simulink model "astr"  (R2017b)
settings: Solver=VariableStepAuto  StartTime=0.0  StopTime=10.0  RelTol=1e-3
undefined symbols (not defined in the file): Cube, mu_s
settings Model: Creator=hazr_sh  LastModifiedBy=shriyahazra

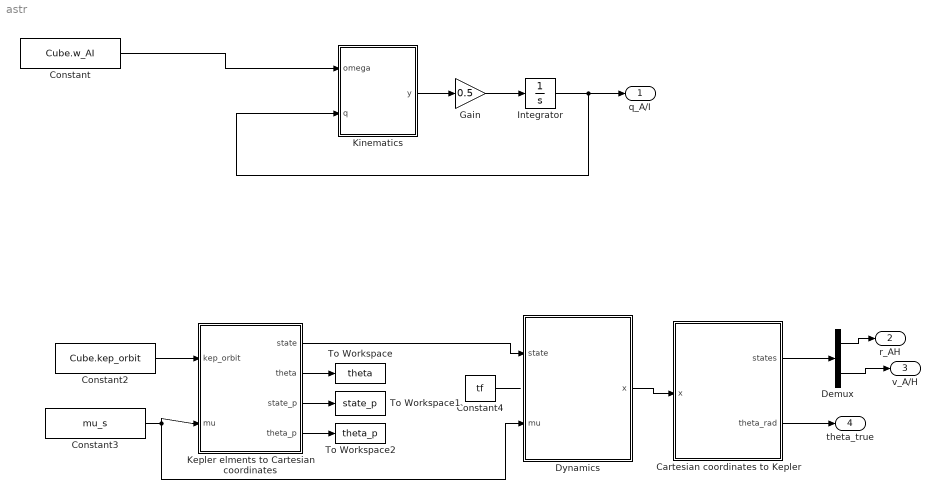
== system astr ==
  Cartesian coordinates to Kepler : MATLAB Function  TreatAsAtomicUnit=on
  Constant : Constant  Value=Cube.w_AI  VectorParams1D=off
  Constant2 : Constant  Value=Cube.kep_orbit  VectorParams1D=off
  Constant3 : Constant  Value=mu_s
  Constant4 : Constant  Value=tf
  Demux : Demux  Outputs=2
  Dynamics : MATLAB Function  TreatAsAtomicUnit=on
  Gain : Gain  Gain=0.5
  Integrator : Integrator  InitialCondition=[0 0 0 0]
  Kepler elments to Cartesian coordinates : MATLAB Function  TreatAsAtomicUnit=on
  Kinematics : MATLAB Function  TreatAsAtomicUnit=on
  To Workspace : ToWorkspace  VariableName=theta  SampleTime=-1
  To Workspace1 : ToWorkspace  VariableName=state_p  SampleTime=-1
  To Workspace2 : ToWorkspace  VariableName=theta_p  SampleTime=-1
  q_A/I : Outport
  r_AH : Outport  Port=2
  v_A/H : Outport  Port=3
  theta_true : Outport  Port=4
  wires:
  Kepler elments to Cartesian coordinates/3(state_p) -> To Workspace1/1
  Kepler elments to Cartesian coordinates/2(theta) -> To Workspace/1
  Dynamics/1(x) -> Cartesian coordinates to Kepler/1(x)
  Gain/1 -> Integrator/1
  Constant2/1 -> Kepler elments to Cartesian coordinates/1(kep_orbit)
  Demux/2 -> v_A/H/1
  Constant4/1 -> ?
  Demux/1 -> r_AH/1
  Cartesian coordinates to Kepler/1(states) -> Demux/1
  Constant3/1 -> Kepler elments to Cartesian coordinates/2(mu), Dynamics/2(mu)
  Cartesian coordinates to Kepler/2(theta_rad) -> theta_true/1
  Kepler elments to Cartesian coordinates/1(state) -> Dynamics/1(state)
  Kepler elments to Cartesian coordinates/4(theta_p) -> To Workspace2/1
  Constant/1 -> Kinematics/1(omega)
  Kinematics/1(y) -> Gain/1
  Integrator/1 -> Kinematics/2(q), q_A/I/1

== matlab function astr/Kinematics ==
  data: omega input; q input; y output
function y = kin(omega, q)
% Quaternion Cross Product
w1 = omega(1);
w2 = omega(2);
w3 = omega(3);

Omega = [0 w3 -w2 w1
         -w3 0 w1 w2
         w2 -w1 0 w3
         -w1 -w2 -w3 0];


y = Omega*q;
end

== matlab function astr/Dynamics ==
  data: state input; x output; mu input
function x  = Propagate_Orbit(state,mu)
%Propagate_Orbit( kepler_orbit, state, mu,tspan)
%This function is to propagate the Kepler orbit subject to only gravity 
%tspan = [0 T+7*24*3600]

% T = 2*pi/kepler_orbit(1,7);
% T = 48*3600;
t0 = 0;
tf = 2*86400;    % Propagate for two days
nsteps = tf/60;

function dx = kepode(t,x)
r = sqrt(x(1)^2 + x(2)^2 + x(3)^2);
dx = [x(5); x(6); x(7); 0; -mu*x(1)/r^3; -mu*x(2)/r^3; -mu*x(3)/r^3; 0];
end

% opts = odeset('Reltol',1e-13,'AbsTol',1e-14,'Stats','on');
% x0 = state;
% [t,x] = ode113(@kepode, tspan, x0, opts);
% plot(t,x)
% legend('x','x''','y','y''','z','z''')
% title('Position and Velocity Components')
tspan = linspace(t0,tf,nsteps);
x0 = state;
x = ode4(@kepode,tspan,x0);

end

== matlab function astr/Cartesian coordinates to Kepler ==
  data: x input; states output; theta_rad output
function [states,theta_rad]  = Cart2kep(x)
%% Cartesian components to Kepler elements
X = [];
R = [];
V = [];
v = [];
H = [];
h = [];
N = [];
n = [];
ee = [];
e = [];
N_xy = [];
theta_rad = [];
theta = [];
p = [];
E_rad = [];
E = [];
M = [];
states = [];

for i = 1:length(x)
    X(i,:) = x(i,1:3);  %state vector
    R(i) = norm(X(i,:));  %magnitude of the X vector

    V(i,:) = x(i,5:7); %velocity vector
    v(i) = norm(V(i,:)); %magnitude of the V vector

    H(i,:) = cross(X(i,:),V(i,:)); %Angular momentum
    h(i) = norm(H(i,:));    %magnitude of the H vector

    s = [0 0 1]';   
    N(i,:) = cross(s,H(i,:));   %Nodal Vector
    n(i) = norm (N(i,:));     %magnitude of the N vector

    ee(i,:) = ((cross(V(i,:),H(i,:))./mu) - X(i,:)./R(i));  %calculating eccentricity vector
    e(i) = norm(ee(i,:));

    N_xy = sqrt (N(1)^2 + N(2)^2);

    theta_rad(i,:) = sign (dot(cross(ee(i,:),X(i,:)),H(i,:))) * acos(dot (X(i,:),ee(i,:))/(R(i)*e(i))); %calculating theta in radians
    theta(i,:) = theta_rad(i,:) * 180/pi;

    p(i,:) = sqrt((1-e(i))/(1+e(i))) * tan(theta_rad(i,:)/2);
    E_rad(i,:) = 2 * atan(p(i,:));
    E(i,:) =  E_rad(i,:) * 180 /pi;  %calculating eccentric anomaly

    M(i,:) = (E_rad(i,:) - e(i) * sin(E_rad(i,:))) * 180 /pi; %calculating mean anomaly
end

states(:,1:3) = X;
states(:,5:7) = V;
states(:,4) = 0;
states(:,8) = 0;
% figure
% hold on
% plot3(x(:,1),x(:,2),x(:,3))
% plot3(0,0,0,'ro')
% axis equal
% title('Orbit of ')
end

== matlab function astr/Kepler elments to Cartesian coordinates ==
  data: kep_orbit input; state output; theta output; mu input; state_p output; theta_p output
function [state,theta,state_p,theta_p] = Kep2cart(kep_orbit,mu)
%% Kepler  elements  to  Cartesian  components
%NASA,2014  data
% kep_orbit(1,1) = 6787746.891;
% kep_orbit(1,2) = 0.000731104;
% kep_orbit(1,3) = 51.68714486*pi /180;
% kep_orbit(1,4) = 127.5486706*pi /180;
% kep_orbit(1,5) = 74.21987137*pi /180;
% kep_orbit(1,6) = 24.06608426*pi /180;


% format  long

Etemp = 0;
deltaE = 1;

while  abs ( deltaE ) > 1e-8 %lower limit for the difference
    E = Etemp + (kep_orbit(1,6)-Etemp + kep_orbit(1,2)*sin (Etemp) ) /(1-kep_orbit(1,2)*cos (Etemp) ) ; %updating E
    deltaE = E-Etemp ; %difference
    Etemp = E; %for next iteration
end

r = kep_orbit(1,1)*(1-kep_orbit(1,2)*cos  (E) );  %position with respect to kepler elements
theta = 2*atan ( sqrt ((1 + kep_orbit(1,2) ) /(1-kep_orbit(1,2) ) )*tan  (E/2) );  %calculating the true anomaly
% true_anomaly = rad2deg(theta);

S = [ ( r*cos  ( theta ) ) 
    ( r*sin  ( theta ) ) ] ; %calculating perifocal co-ordinates

l1 = cos (kep_orbit(1,4))*cos (kep_orbit(1,5))-sin  (kep_orbit(1,4))*sin  (kep_orbit(1,5))*cos ( kep_orbit(1,3) ) ;
l2 =-cos (kep_orbit(1,4))*sin (kep_orbit(1,5))-sin  (kep_orbit(1,4))*cos  (kep_orbit(1,5))*cos ( kep_orbit(1,3) ) ;
m1 = sin (kep_orbit(1,4))*cos (kep_orbit(1,5)) + cos  (kep_orbit(1,4))*sin  (kep_orbit(1,5))*cos ( kep_orbit(1,3) ) ;
m2 =-sin (kep_orbit(1,4))*sin (kep_orbit(1,5)) + cos  (kep_orbit(1,4))*cos  (kep_orbit(1,5))*cos ( kep_orbit(1,3) ) ;
n1 = sin  (kep_orbit(1,5))*sin  ( kep_orbit(1,3) ) ;
n2 = cos (kep_orbit(1,5))*sin  ( kep_orbit(1,3) ) ;

H = sqrt (mu*kep_orbit(1,1)*(1-kep_orbit(1,2) ^2) ) ; %calculating angular momentum

L = [ l1  l2
      m1 m2
      n1 n2 ] ;

X = L*S ;  %calculating the state vector
V = [ (mu/H*(-l1*sin  ( theta ) + l2*( kep_orbit(1,2) + cos ( theta ) ) ) )    %calculating the velocity vector
      (mu/H*(-m1*sin  ( theta ) + m2*( kep_orbit(1,2) + cos ( theta ) ) ) )
      (mu/H*(-n1*sin  ( theta ) + n2*( kep_orbit(1,2) + cos ( theta ) ) ) ) ] ;
  
state = [X;0;V;0];
% Cartesian = { 'x ' ;  'y ' ;  ' z ' ;  ' xdot ' ;  ' ydot ' ;  ' zdot ' };
% Values = [X(1) ; X(2) ; X(3) ; V(1) ; V(2) ; V(3) ] ;
% T = table ( Cartesian ,  Values );


%% State at pericentre

% format  long
E_p=0;

r_p = kep_orbit(1,1)*(1-kep_orbit(1,2)*cos  (E_p) );  %position with respect to kepler elements
theta_p = 2*atan ( sqrt ((1 + kep_orbit(1,2) ) /(1-kep_orbit(1,2) ) )*tan  (E_p/2) );  %calculating the true anomaly
% true_anomaly_p = rad2deg(theta_p);

S_p = [ ( r_p*cos  ( theta_p ) ) 
    ( r_p*sin  ( theta_p ) ) ] ; %calculating perifocal co-ordinates

l1_p = cos (kep_orbit(1,4))*cos (kep_orbit(1,5))-sin  (kep_orbit(1,4))*sin  (kep_orbit(1,5))*cos ( kep_orbit(1,3) ) ;
l2_p =-cos (kep_orbit(1,4))*sin (kep_orbit(1,5))-sin  (kep_orbit(1,4))*cos  (kep_orbit(1,5))*cos ( kep_orbit(1,3) ) ;
m1_p = sin (kep_orbit(1,4))*cos (kep_orbit(1,5)) + cos  (kep_orbit(1,4))*sin  (kep_orbit(1,5))*cos ( kep_orbit(1,3) ) ;
m2_p =-sin (kep_orbit(1,4))*sin (kep_orbit(1,5)) + cos  (kep_orbit(1,4))*cos  (kep_orbit(1,5))*cos ( kep_orbit(1,3) ) ;
n1_p = sin  (kep_orbit(1,5))*sin  ( kep_orbit(1,3) ) ;
n2_p = cos (kep_orbit(1,5))*sin  ( kep_orbit(1,3) ) ;

H_p = sqrt (mu*kep_orbit(1,1)*(1-kep_orbit(1,2) ^2) ) ; %calculating angular momentum

L_p = [ l1_p  l2_p
      m1_p m2_p
      n1_p n2_p ] ;

X_p = L_p*S_p ;  %calculating the state vector
V_p = [ (mu/H_p*(-l1_p*sin  ( theta_p ) + l2_p*( kep_orbit(1,2) + cos ( theta_p ) ) ) )    %calculating the velocity vector
      (mu/H_p*(-m1_p*sin  ( theta_p ) + m2_p*( kep_orbit(1,2) + cos ( theta_p ) ) ) )
      (mu/H_p*(-n1_p*sin  ( theta_p ) + n2_p*( kep_orbit(1,2) + cos ( theta_p ) ) ) ) ] ;
  
state_p = [X_p;0;V_p;0];

end
